simulink library "INT_GlwLmp_DD"  (R2016b)
settings: Solver=VariableStepAuto  StartTime=0.0  StopTime=10.0  RelTol=1e-3
settings Model: Creator=liutao  LastModifiedBy=liutao

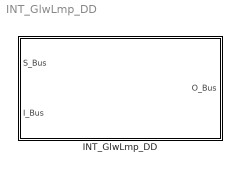
== system INT_GlwLmp_DD ==
  INT_GlwLmp_DD : Subsystem

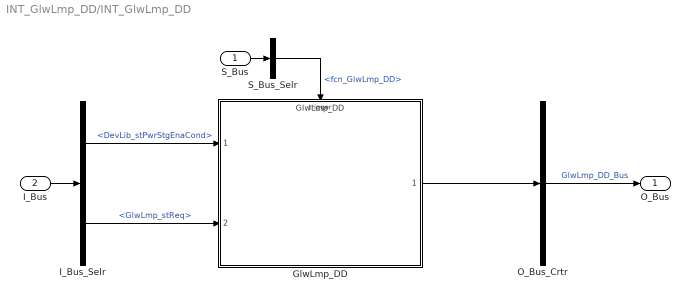
== system INT_GlwLmp_DD/INT_GlwLmp_DD ==
  S_Bus : Inport
  I_Bus : Inport  Port=2
  GlwLmp_DD : ModelReference  ModelNameDialog=GlwLmp_DD  SimulationMode=Normal  ModelReferenceVersion=1.9  TriggerPortName=function  TriggerPortTriggerType=function-call  TriggerPortStatesWhenEnabling=held
  I_Bus_Selr : BusSelector  OutputSignals=DevLib_stPwrStgEnaCond,GlwLmp_stReq
  O_Bus_Crtr : BusCreator  Inputs=1
  S_Bus_Selr : BusSelector  OutputSignals=fcn_GlwLmp_DD
  O_Bus : Outport
  wires:
  S_Bus_Selr/1 -> GlwLmp_DD/Trigger  "<fcn_GlwLmp_DD>"
  S_Bus/1 -> S_Bus_Selr/1
  I_Bus/1 -> I_Bus_Selr/1
  I_Bus_Selr/1 -> GlwLmp_DD/1  "<DevLib_stPwrStgEnaCond>"
  I_Bus_Selr/2 -> GlwLmp_DD/2  "<GlwLmp_stReq>"
  O_Bus_Crtr/1 -> O_Bus/1  "GlwLmp_DD_Bus"
  GlwLmp_DD/1 -> O_Bus_Crtr/1
